simulink model "PI_controller"  (R2020b)
settings: Solver=VariableStepAuto  StartTime=0.0  StopTime=10  RelTol=1e-3
undefined symbols (not defined in the file or in its folder): ki, kp
settings Model: DataDictionary=Problem3_data.sldd  Creator=ASUS  LastModifiedBy=ASUS
settings DataIOCC: SaveOutput=off  SaveTime=off

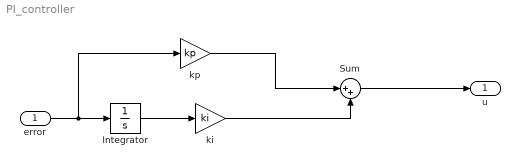
== system PI_controller ==
  error : Inport  OutDataTypeStr=double  PortDimensions=1  SampleTime=0
  Integrator : Integrator
  Sum : Sum  Inputs=|++
  ki : Gain  Gain=ki
  kp : Gain  Gain=kp
  u : Outport  OutDataTypeStr=double  PortDimensions=1  SampleTime=0
  wires:
  Sum/1 -> u/1
  error/1 -> Integrator/1, kp/1
  kp/1 -> Sum/1
  Integrator/1 -> ki/1
  ki/1 -> Sum/2
